simulink library "DQN_Lib"  (R2023b)
settings: Solver=VariableStepAuto  StartTime=0.0  StopTime=10.0  RelTol=1e-3
undefined symbols (not defined in the file): ACDC3, HRM, La, N, R, Ra, sps_AC, SYS, Ts, Ts_dqn, Ts_Power, w, Ws
libraries: DQN_Lib_bak x7
(part 1 of 3)
settings Model: Creator=Robert  LastModifiedBy=rober
settings DebuggingCC: UnconnectedInputMsg=warning  UnconnectedOutputMsg=warning  UnconnectedLineMsg=warning
settings ModelReferenceCC: EnableRefExpFcnMdlSchedulingChecks=on
settings RTWCC: DLArmComputeVersion=19.05

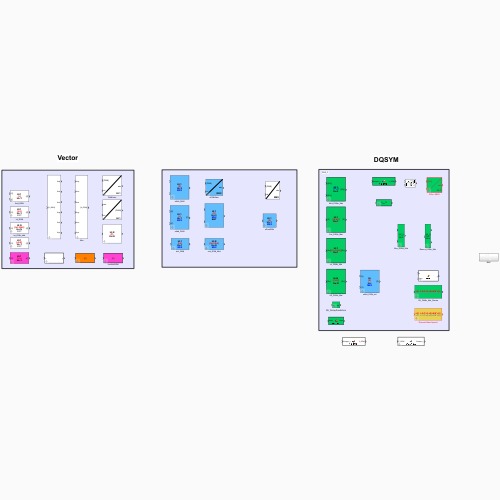
[thumbnail: Simulink's stored preview of the top-level diagram]
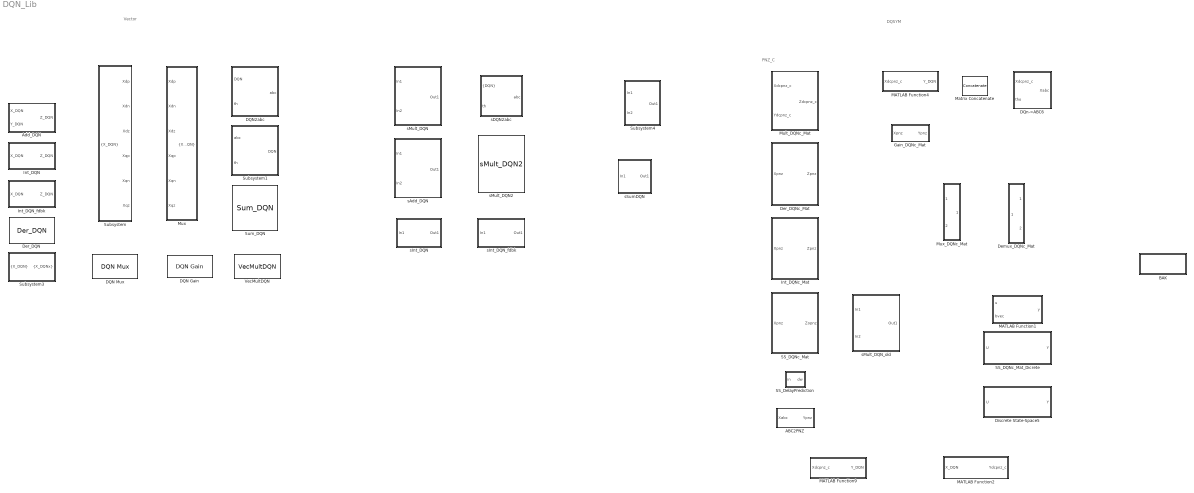
== system DQN_Lib ==
  note: PNZ_C
  note: DQSYM
  note: Vector
  ABC2PNZ : MATLAB Function  TreatAsAtomicUnit=on  SystemSampleTime=Ts
  Add_DQN : Subsystem  mask{HrmOrd=1, chkHrmLst=off, HrmLst=[1]}
      mask prompts: HrmOrd "Harmonic order:"; chkHrmLst "Only specific harmonics"; HrmLst "Harmonic list:"
      mask Callback chkHrmLst:
      | EMT = get_param(gcb,'chkHrmLst');
      | 
      | if(strcmp(EMT,'on'))
      |    set_param(gcb,'MaskVisibilities',{'on','on','on'});
      | else
      |    set_param(gcb,'MaskVisibilities',{'on','on','off'});
      | end
      mask Display:
      | %plot([0 1])
      | port_label('input',1,'{X}');
      | port_label('input',2,'{Y}');
      | port_label('output',1,'{Z}');
      | 
      | 
      | 
      | harm = get_param(gcb, 'HrmOrd');
      | disp(['{\color{black}\bf\fontsize{12}Hi:',(harm),'}',newline,'{\color{red}\bf\fontsize{12}\{+\}}',newline,'{\color{black}\bf\fontsize{12}Ho:',(harm),'}'], 'texmode','on');
  BAK : Subsystem
  DQN Gain : DQN_Lib_bak/DQN Gain  H=1  Rvec=[]
  DQN Mux : DQN_Lib_bak/DQN Mux  N=1
  DQN2abc : Subsystem  mask{HrmOrd=1}
      mask prompts: HrmOrd "Harmonic order:"
      mask Display:
      | plot([0 1], [0,1])
      | port_label('input',1,'{DQN}');
      | port_label('input',2,'wt');
      | port_label('output',1,'abc');
      | 
      | 
      | 
      | harm = get_param(gcb, 'HrmOrd');
      | %disp([newline,'{\bf\fontsize{12}H=',harm,'}'], 'texmode','on');
      | text(.95,.05,[newline,'{\bf\fontsize{12}H=',harm,'}'], 'horizontalAlignment', 'right', 'verticalAlignment','bottom','texmode','on')
  DQn->ABC6 : MATLAB Function  TreatAsAtomicUnit=on  mask{N=1}
      mask prompts: N "Harmonic order:"
  Demux_DQNc_Mat : Subsystem  mask{nrOut=2}
      mask prompts: nrOut "Number of outputs [{C}]"
      mask init:
      | if(isempty(nrOut))
      |     Simulink.SubSystem.deleteContents(gcb);
      | else
      | 
      |     IndexOptionArray = cell(2,1);
      |     IndexOptionArray(1) = {'Select all'           };
      |     IndexOptionArray(2) = {'Index vector (dialog)'};
      | 
      |     PortHandles = get_param(gcb,'PortHandles');
      | 
      |     lenOut = length(PortHandles.Outport);
      | 
      |     if(nrOut ~= lenOut) % Important to avoid reinitialization of the block!
      | 
      |         Simulink.SubSystem.deleteContents(gcb);
      | 
      |         add_block('built-in/Inport',[gcb,strcat('/In',num2str(1))]);
      |         set_param([gcb,strcat('/In',num2str(1))],'position' , [50,65+1*50,90,85+1*50]);
      | 
      |         for i = 1 : nrOut
      |             add_block('simulink/Signal Routing/Selector',[gcb,strcat('/Sel',num2str(i))],...
      |                 'IndexOptionArray',IndexOptionArray,...
      |                 'NumberOfDimensions','2',...
      |                 'IndexOptions','Index vector (dialog),Select all',...
      |                 'Indices',strcat(num2str((i-1)*3+1),':',num2str((i-1)*3+3),', 1') ...
      |                 );
      |             set_param([gcb,strcat('/Sel',num2str(i))],'position' , [450,65+i*50,490,85+i*50])
      | 
      | 
      |             add_block('built-in/Outport',[gcb,strcat('/Out',num2str(i))]);
      |             set_param([gcb,strcat('/Out',num2str(i))],'position' , [750,65+i*50,790,85+i*50]);
      | 
      |             add_line(gcb,strcat('In',num2str(1),'/1'),  strcat('Sel',num2str(i),'/1'),'autorouting','on');
      |             add_line(gcb,strcat('Sel',num2str(i),'/1'), strcat('Out',num2str(i),'/1'),'autorouting','on');
      |         end
      | 
      |     end
      | 
      | end
      mask Display: disp(['{\color{red}\bf\fontsize{12}} [\{X_C\}]',newline,' DE-',newline,' MUX'], 'texmode','on');
  Der_DQN : DQN_Lib_bak/Der_DQN  HrmOrd=1  FreqRad=2*pi*50  Ts=0  EMT=on  sw_soft=on  chkHrmLst=off  HrmLst=[1]
  Der_DQNc_Mat : MATLAB Function  TreatAsAtomicUnit=on  mask{Ts=50e-6, N=1, w=2*pi*50, EMT=on, sw_soft=on}
      mask prompts: Ts "Time step (s):"; N "Harmonic order:"; w "Angular frequency [1/rad]:"; sw_soft "Soft start"
  Discrete State-Space5 : Subsystem  mask{A=sps_AC.A, B=sps_AC.B, C=sps_AC.C, D=sps_AC.D, InitVec=sps_AC.x0, dt=Ts_Power, DQSYM=on, N=HRM, Ws=w}
      mask prompts: InitVec "Initial condition:"; dt "Time step (s):"; N "Harmonic number:"; Ws "Angular frequency (1/rad):"
      mask init:
      | % I = eye(size(A,1));
      | % INVR = I/(I-A*dt/2);
      | % Ad1 = INVR*(I+A*dt/2);
      | % Bd1 = INVR*B*dt/2;
      | % Cd1 = C*Ad1;
      | % Dd11 = C*INVR*B*dt/2+D;
      | % Dd12 = C*INVR*B*dt/2;
      | 
      |     I = eye(size(A,1));
      |     INVR = I/(I-A*dt/2);
      |     Ad1 = INVR*(I+A*dt/2);
      |     Bd1 = INVR*B;
      |     Cd1 = C*INVR*dt;
      |     Dd1 = Cd1*B/2 + D;
      | 
      | DQSYM = get_param(gcb,'DQSYM');
      | 
      | comp = 0;
      | 
      | if(strcmp(DQSYM,'on'))
      | 
      | %Calculating the PNZ matrices
      | 
      |     a = -0.5+0.866i;
      |     a2 = -0.5-0.866i;
      |     Sas = [1,a,a2;1,a2,a;1,1,1]/3;
      | 
      |     arows = size(Ad1,1)/3; %signal size
      |     acols = size(Ad1,2)/3; %signal size
      | 
      |     brows = size(Bd1,1)/3; %signal size
      |     bcols = size(Bd1,2)/3; %signal size
      | 
      |     crows = size(Cd1,1)/3; %signal size
      |     ccols = size(Cd1,2)/3; %signal size
      | 
      |     d1rows = size(Dd1,1)/3; %signal size
      |     d1cols = size(Dd1,2)/3; %signal size
      | 
      |     %%%%%%%%%%%%%%%%%%%%%%% Check for inconsistencies  %%%%%%%%%%%%%%%%%%%%%%%
      | 
      |     szMatA = size(A,1);
      |     iL = eye(szMatA);
      |     szMatiL = size(iL,1);
      | 
      |     if(szMatiL ~= szMatA || size(A,1) ~= size(A,2) || size(iL,1) ~= size(iL,2))
      |         error('[Int_DQN_Mat/swFeedback] check matrix A size!');
      |     end
      | 
      |     if(arows ~= brows || acols ~= ccols || crows ~= d1rows || bcols ~= d1cols)
      |         error('[Int_DQN_Mat/Initialize] the sizes of the state-space matrices!');
      |     end
      | 
      |     %%%%%%%%%%%%%%%%%%%%%%%%%%%%%%%%%%%%%%%%%%%%%%%%%%%%%%%%%%%%%%%
      | 
      | 
      |     %%%%%%%%%%%%%%%%%%%%%%% A --> Bpnz %%%%%%%%%%%%%%%%%%%%%%%
      |     Adc = complex(zeros(3*arows,3*acols));
      | 
      |     for i = 1 : arows
      |         for j = 1 : acols
      |             Adc((1:3) + (i-1)*3,(1:3) + (j-1)*3) = Sas*Ad1((1:3) + (i-1)*3,(1:3) + (j-1)*3)/Sas;
      |             %Adc((1:3) + (i-1)*3,(1:3) + (j-1)*3) = diag(diag(real(Adc((1:3) + (i-1)*3,(1:3) + (j-1)*3))));
      |             %Adc((1:3) + (i-1)*3,(1:3) + (j-1)*3) = diag(diag((Adc((1:3) + (i-1)*3,(1:3) + (j-1)*3))));
      | 
      |         end
      |     end
      |     %%%%%%%%%%%%%%%%%%%%%%%%%%%%%%%%%%%%%%%%%%%%%%%%%%%%%%%%%%%%%%%
      | 
      |     %%%%%%%%%%%%%%%%%%%%%%% B --> Bpnz %%%%%%%%%%%%%%%%%%%%%%%
      | 
      |     Bdc = complex(zeros(3*brows,3*bcols));
      | 
      |     for i = 1 : brows
      |         for j = 1 : bcols
      |             Bdc((1:3) + (i-1)*3,(1:3) + (j-1)*3) = Sas*Bd1((1:3) + (i-1)*3,(1:3) + (j-1)*3)/Sas;
      |             %Bdc((1:3) + (i-1)*3,(1:3) + (j-1)*3) = diag(diag(real(Bdc((1:3) + (i-1)*3,(1:3) + (j-1)*3))));
      |             %Bdc((1:3) + (i-1)*3,(1:3) + (j-1)*3) = diag(diag((Bdc((1:3) + (i-1)*3,(1:3) + (j-1)*3))));
      | 
      |         end
      |     end
      |     %%%%%%%%%%%%%%%%%%%%%%%%%%%%%%%%%%%%%%%%%%%%%%%%%%%%%%%%%%%%%%%
      | 
      |     %%%%%%%%%%%%%%%%%%%%%%% C --> Cpnz %%%%%%%%%%%%%%%%%%%%%%%
      | 
      |     Cdc = complex(zeros(3*crows,3*ccols));
      | 
      |     for i = 1 : crows
      |         for j = 1 : ccols
      |             Cdc((1:3) + (i-1)*3,(1:3) + (j-1)*3) = Sas*Cd1((1:3) + (i-1)*3,(1:3) + (j-1)*3)/Sas;
      |             %Cdc((1:3) + (i-1)*3,(1:3) + (j-1)*3) = diag(diag(real(Cdc((1:3) + (i-1)*3,(1:3) + (j-1)*3))));
      |             %Cdc((1:3) + (i-1)*3,(1:3) + (j-1)*3) = diag(diag((Cdc((1:3) + (i-1)*3,(1:3) + (j-1)*3))));
      |         end
      |     end
      |     %%%%%%%%%%%%%%%%%%%%%%%%%%%%%%%%%%%%%%%%%%%%%%%%%%%%%%%%%%%%%%%
      | 
      |     
      |     %%%%%%%%%%%%%%%%%%%%%%% D1 --> Cpnz %%%%%%%%%%%%%%%%%%%%%%%
      | 
      |     Ddc = complex(zeros(3*d1rows,3*d1cols));
      | 
      |     for i = 1 : d1rows
      |         for j = 1 : d1cols
      |             Ddc((1:3) + (i-1)*3,(1:3) + (j-1)*3) = Sas*Dd1((1:3) + (i-1)*3,(1:3) + (j-1)*3)/Sas;
      |             %Ddc1((1:3) + (i-1)*3,(1:3) + (j-1)*3) = diag(diag(real(Ddc1((1:3) + (i-1)*3,(1:3) + (j-1)*3))));
      |             %Ddc((1:3) + (i-1)*3,(1:3) + (j-1)*3) = diag(diag((Ddc((1:3) + (i-1)*3,(1:3) + (j-1)*3))));
      |         end
      |     end
      |     %%%%%%%%%%%%%%%%%%%%%%%%%%%%%%%%%%%%%%%%%%%%%%%%%%%%%%%%%%%%%%%
      | 
      |     Adc(abs(Adc)<2*eps) = 0;
      |     Bdc(abs(Bdc)<2*eps) = 0;
      |     Cdc(abs(Cdc)<2*eps) = 0;
      |     Ddc(abs(Ddc)<2*eps) = 0;
      | 
      |     InitVec_c = complex(zeros(brows*3,N+1));
      | 
      | 
      |     if(~isempty(InitVec))
      |         if(mod(numel(InitVec),3)~=0) 
      |             warning('[SS_DQNc_Mat] InitVec with wrong size --> needs to be a multiple of 3!'); 
      | 
      |         else
      |             for k = 1 : numel(InitVec)/3
      |                 InitVec_c((k-1)*3+1:(k-1)*3+3,1) = Sas*InitVec((k-1)*3+1:(k-1)*3+3)*exp(+1i*Ws*dt);
      |             end
      |         end
      |     end
      | 
      |     InitVec = InitVec_c;
      | 
      | 
      |     Ad1 = Adc;
      |     Bd1 = Bdc;
      |     Cd1 = Cdc;
      |     Dd1 = Ddc;
      | 
      |     comp = -1i*Ws*dt;
      | 
      | end
      settings: LibrarySourceBlock=|
      | spsSynchronousMachineModel/Discrete robust/State Space Model/Discretize
      | BE or Tustin
      mask Callback DQSYM:
      | EMT = get_param(gcb,'DQSYM');
      | 
      | if(strcmp(EMT,'on'))
      |    set_param(gcb,'MaskVisibilities',{'on','on','on','on','on','on','on','on','on'});
      | else
      |    set_param(gcb,'MaskVisibilities',{'on','on','on','on','on','on','on','off','off'});
      | end
      mask Display: disp(['{\color{red}\bf\fontsize{12}x(t) = Ad*x(t-dt)+Bd*u(t)}',newline,'{\color{gray}\bf\fontsize{12}y(t) = Cd*x(t-dt)+Dd*u(t)}'], 'texmode','on');
  Gain_DQNc_Mat : MATLAB Function  TreatAsAtomicUnit=on  mask{Rabc=[R zeros(3,3); zeros(3,3) R], HRM=N, chkInv=off}
      mask prompts: Rabc "Line matrix [3x3]:"; HRM "Harmonic order:"; chkInv "Invert"
  Int_DQN : Subsystem  mask{HrmOrd=1, FreqRad=2*pi*50, TimeStep=50e-6, Init=zeros(1,6), EMT=on, chkHrmLst=off, HrmLst=[1]}
      mask prompts: HrmOrd "Harmonic order:"; FreqRad "Angular frequency (rad/s);"; TimeStep "Time step (s):"; Init "DC init [1x6]:"; EMT "Enable EMT"; chkHrmLst "Only specific harmonics"; HrmLst "Harmonic list:"
      mask Callback chkHrmLst:
      | EMT = get_param(gcb,'chkHrmLst');
      | 
      | if(strcmp(EMT,'on'))
      |    set_param(gcb,'MaskVisibilities',{'on','on','on','on','on','on','on'});
      | else
      |    set_param(gcb,'MaskVisibilities',{'on','on','on','on','on','on','off'});
      | end
      mask Display:
      | %plot([0 1])
      | port_label('input',1,'{X}');
      | port_label('output',1,'{Z}');
      | 
      | harm = get_param(gcb, 'HrmOrd');
      | 
      | if(numel(get_param(gcb, 'EMT'))==2)
      |     disp(['{\color{black}\bf\fontsize{12}Hi:',(harm),'}',newline,'{\color{red}\bf\fontsize{12}\{Int\}}',newline,'{\color{black}\bf\fontsize{12}Ho:',(harm),'}',newline,'{\color{gray}\bf\fontsize{12}EMT}'], 'texmode','on');
      | else
      |     disp(['{\color{black}\bf\fontsize{12}Hi:',(harm),'}',newline,'{\color{red}\bf\fontsize{12}\{Int\}}',newline,'{\color{black}\bf\fontsize{12}Ho:',(harm),'}'], 'texmode','on');
      | end
  Int_DQN_fdbk : Subsystem  mask{HrmOrd=N, FreqRad=Ws, TimeStep=Ts_dqn, swFeed=on, R=Ra, iL=1/La}
      mask prompts: HrmOrd "Harmonic order:"; FreqRad "Angular frequency (rad/s);"; TimeStep "Time step (s):"; swFeed "Enable feedback"; R "Feedback parameter (Kr):"; iL "Integrator parameter (Kl):"
      mask Callback swFeed:
      | EMT = get_param(gcb,'swFeed');
      | 
      | if(strcmp(EMT,'on'))
      |    set_param(gcb,'MaskVisibilities',{'on','on','on','on','on','on'});
      | else
      |    set_param(gcb,'MaskVisibilities',{'on','on','on','on','off','off'});
      | end
      mask Display:
      | %plot([0 1])
      | port_label('input',1,'{X}');
      | port_label('output',1,'{Z}');
      | 
      | harm = get_param(gcb, 'HrmOrd');
      | disp(['{\color{black}\bf\fontsize{12}Hi:',(harm),'}',newline,'{\color{red}\bf\fontsize{12}\{Int-fdbk\}}',newline,'{\color{black}\bf\fontsize{12}Ho:',(harm),'}',newline,'{\color{gray}\bf\fontsize{12}EMT}'], 'texmode','on');
  Int_DQNc_Mat : MATLAB Function  TreatAsAtomicUnit=on  mask{N=1, dt=50e-6, w=2*pi*50, InitInt=zeros(3,1), swFeed=on, R=eye(3), iL=eye(3)}
      mask prompts: N "Order number:"; dt "Time step (s):"; w "Angular frequency (1/rad):"; InitInt "Initial conditions DC [3x1]:"; swFeed "Enable feedback"; R "Feedback parameter (Kr {abc}):"; iL "Feedback parameter (Ki {abc}):"
  MATLAB Function1 : MATLAB Function  TreatAsAtomicUnit=on  mask{Ad=ACDC3.Adiscrete, Bd=ACDC3.Bdiscrete, Cd=ACDC3.Cdiscrete, Dd=ACDC3.Ddiscrete, InitVec=ACDC3.x0, dt=Ts_Power, nsw=6}
      mask prompts: Ad "A"; Bd "B"; Cd "C"; Dd "D"; InitVec "Initial values:"; dt "Time step (s):"; nsw "Number of switches:"
  MATLAB Function2 : MATLAB Function  TreatAsAtomicUnit=on  mask{N=HRM}
      mask prompts: N "Harmonic order:"
  MATLAB Function4 : MATLAB Function  TreatAsAtomicUnit=on
  MATLAB Function9 : MATLAB Function  TreatAsAtomicUnit=on
  Matrix Concatenate : Concatenate  Mode=Multidimensional array  ConcatenateDimension=2
  Mult_DQNc_Mat : MATLAB Function  TreatAsAtomicUnit=on  mask{N=1, HrmDbl=on}
      mask prompts: N "Harmonic order:"; HrmDbl "Double Harmonic"
  Mux : Subsystem  mask{N=1}
      mask prompts: N "Harmonic order:"
  Mux_DQNc_Mat : Subsystem  mask{nrInp=2}
      mask prompts: nrInp "Number of inputs [{C}]"
      mask init:
      | %blocks = find_system(gcb,'LookUnderMasks','on','FollowLinks','on')
      | %set_param(gcb, 'MaskSelfModifiable', 'on');
      | 
      | % if(SSM == [])
      | %     Simulink.SubSystem.deleteContents(gcb);
      | % else
      | 
      | if(isempty(nrInp))
      |     Simulink.SubSystem.deleteContents(gcb);
      | else
      | 
      |     nrOut = 1;
      | 
      | 
      | PortHandles = get_param(gcb,'PortHandles');
      | lenInp = length(PortHandles.Inport);
      | lenOut = length(PortHandles.Inport);
      | 
      | if(nrInp ~= lenInp)
      |     %disp('ENTERED')
      |     Simulink.SubSystem.deleteContents(gcb);
      | %     add_block('simulink/Continuous/State-Space', [gcb,'/ss_block'], 'A','SS.A', 'B','SS.B', 'C','SS.C', 'D','SS.D', 'X0','X0')
      | %     set_param([gcb,'/ss_block'],'position' , [350,100,450,150])
      | 
      | 
      | 
      |         add_block('simulink/Math Operations/Matrix Concatenate',[gcb,'/Mux'], 'NumInputs',num2str(nrInp), 'ConcatenateDimension',num2str(1));
      |         set_param([gcb,'/Mux'],'position' , [200,100,250,100+nrInp*50])
      |         
      | %         add_block('built-in/Demux',[gcb,'/Demux'], 'Outputs',num2str(nrOut));
      | %         set_param([gcb,'/Demux'],'position' , [500,100,550,100+nrOut*50])
      | 
      | 
      |         for i = 1 : nrInp
      |             add_block('built-in/Inport',[gcb,strcat('/In',num2str(i))]);
      |             set_param([gcb,strcat('/In',num2str(i))],'position' , [50,65+i*50,90,85+i*50]);
      |             add_line(gcb,strcat('In',num2str(i),'/1'),strcat('Mux/',num2str(i)),'autorouting','on');
      |         end
      | 
      |         for i = 1 : nrOut
      |             add_block('built-in/Outport',[gcb,strcat('/Out',num2str(i))]);
      |             set_param([gcb,strcat('/Out',num2str(i))],'position' , [750,65+i*50,790,85+i*50]);
      |             add_line(gcb,strcat('Mux/',num2str(i)), strcat('Out',num2str(i),'/1'),'autorouting','on');
      |         end
      | 
      | 
      | %     add_line(gcb, 'Mux/1', 'ss_block/1')
      | %     add_line(gcb, 'ss_block/1', 'Demux/1')
      | 
      | end
      | 
      | end
      mask Display: disp(['{\color{red}\bf\fontsize{12}} [\{X_C\}]',newline,' MUX'], 'texmode','on');
  SS_DQNc_Mat : MATLAB Function  TreatAsAtomicUnit=on  mask{N=N, A=[], B=[], C=[], D=[], dt=50e-6, w=2*pi*50, x0=[], stNames=[]}
      mask prompts: N "Order number:"; dt "Time step (s):"; w "Angular frequency (1/rad):"; x0 "Initial conditions:"; stNames "State names:"
      mask init:
      | szA = size(A,1);
      | 
      | [~, I] = sort(stNames(1:szA));
      | 
      | 
      | A = A(I,I);
      | B = B(I,:);
      | C = -C(:,I);
      | D = D;
      | 
      | x0 = x0(I,:);
  SS_DQNc_Mat_Dicrete : Subsystem  mask{A=SYS.A, B=SYS.B, C=SYS.C, D=SYS.D, InitVec=SYS.x0, dt=Ts, N=N, Ws=2*pi*50}
      mask prompts: InitVec "Initial condition:"; dt "Time step (s):"; N "Harmonic order:"; Ws "Angular frequency (rad/s):"
      mask init:
      | I = eye(size(A,1));
      |     
      |     INVR = I/(I-A*dt/2);
      |     
      |     Ad = INVR*(I+A*dt/2);
      |     
      |     Bd = INVR*B;
      |     
      |     Cd = C*INVR*dt;
      |     
      |     Dd = Cd*B/2;
      | 
      |     dt2 = dt/2;
      | 
      |     a = -0.5+0.866i;
      |     a2 = -0.5-0.866i;
      |     Sas = [1,a,a2;1,a2,a;1,1,1]/3;
      | 
      |     arows = size(Ad,1)/3; %signal size
      |     acols = size(Ad,2)/3; %signal size
      | 
      |     brows = size(Bd,1)/3; %signal size
      |     bcols = size(Bd,2)/3; %signal size
      | 
      |     crows = size(Cd,1)/3; %signal size
      |     ccols = size(Cd,2)/3; %signal size
      | 
      |     drows = size(Dd,1)/3; %signal size
      |     dcols = size(Dd,2)/3; %signal size
      | 
      |     %%%%%%%%%%%%%%%%%%%%%%% Check for inconsistencies  %%%%%%%%%%%%%%%%%%%%%%%
      | 
      |     szMatA = size(A,1);
      |     iL = eye(szMatA);
      |     szMatiL = size(iL,1);
      | 
      |     if(szMatiL ~= szMatA || size(A,1) ~= size(A,2) || size(iL,1) ~= size(iL,2))
      |         error('[Int_DQN_Mat/swFeedback] check matrix A size!');
      |     end
      | 
      |     if(arows ~= brows || acols ~= ccols || crows ~= drows || bcols ~= dcols)
      |         error('[Int_DQN_Mat/Initialize] the sizes of the state-space matrices!');
      |     end
      | 
      |     %%%%%%%%%%%%%%%%%%%%%%%%%%%%%%%%%%%%%%%%%%%%%%%%%%%%%%%%%%%%%%%
      | 
      |     %%%%%%%%%%%%%%%%%%%%%%% A --> Bpnz %%%%%%%%%%%%%%%%%%%%%%%
      |     Adc = complex(zeros(3*arows,3*acols));
      | 
      |     for i = 1 : arows
      |         for j = 1 : acols
      |             Adc((1:3) + (i-1)*3,(1:3) + (j-1)*3) = Sas*Ad((1:3) + (i-1)*3,(1:3) + (j-1)*3)/Sas;
      |             %Adc((1:3) + (i-1)*3,(1:3) + (j-1)*3) = diag(diag(real(Adc((1:3) + (i-1)*3,(1:3) + (j-1)*3))));
      |         end
      |     end
      |     %%%%%%%%%%%%%%%%%%%%%%%%%%%%%%%%%%%%%%%%%%%%%%%%%%%%%%%%%%%%%%%
      | 
      |     %%%%%%%%%%%%%%%%%%%%%%% B --> Bpnz %%%%%%%%%%%%%%%%%%%%%%%
      | 
      |     Bdc = complex(zeros(3*brows,3*bcols));
      | 
      |     for i = 1 : brows
      |         for j = 1 : bcols
      |             Bdc((1:3) + (i-1)*3,(1:3) + (j-1)*3) = Sas*Bd((1:3) + (i-1)*3,(1:3) + (j-1)*3)/Sas;
      |             %Bdc((1:3) + (i-1)*3,(1:3) + (j-1)*3) = diag(diag(real(Bdc((1:3) + (i-1)*3,(1:3) + (j-1)*3))));
      |         end
      |     end
      |     %%%%%%%%%%%%%%%%%%%%%%%%%%%%%%%%%%%%%%%%%%%%%%%%%%%%%%%%%%%%%%%
      | 
      |     %%%%%%%%%%%%%%%%%%%%%%% C --> Cpnz %%%%%%%%%%%%%%%%%%%%%%%
      | 
      |     Cdc = complex(zeros(3*crows,3*ccols));
      | 
      |     for i = 1 : crows
      |         for j = 1 : ccols
      |             Cdc((1:3) + (i-1)*3,(1:3) + (j-1)*3) = Sas*Cd((1:3) + (i-1)*3,(1:3) + (j-1)*3)/Sas;
      |             %Cdc((1:3) + (i-1)*3,(1:3) + (j-1)*3) = diag(diag(real(Cdc((1:3) + (i-1)*3,(1:3) + (j-1)*3))));
      |         end
      |     end
      |     %%%%%%%%%%%%%%%%%%%%%%%%%%%%%%%%%%%%%%%%%%%%%%%%%%%%%%%%%%%%%%%
      | 
      |     %%%%%%%%%%%%%%%%%%%%%%% C --> Cpnz %%%%%%%%%%%%%%%%%%%%%%%
      | 
      |     Ddc = complex(zeros(3*drows,3*dcols));
      | 
      |     for i = 1 : drows
      |         for j = 1 : dcols
      |             Ddc((1:3) + (i-1)*3,(1:3) + (j-1)*3) = Sas*Dd((1:3) + (i-1)*3,(1:3) + (j-1)*3)/Sas;
      |             %Ddc((1:3) + (i-1)*3,(1:3) + (j-1)*3) = diag(diag(real(Ddc((1:3) + (i-1)*3,(1:3) + (j-1)*3))));
      |         end
      |     end
      |     %%%%%%%%%%%%%%%%%%%%%%%%%%%%%%%%%%%%%%%%%%%%%%%%%%%%%%%%%%%%%%%
      | 
      | 
      | 
      |     Adc(abs(Adc)<2*eps) = 0;
      |     Bdc(abs(Bdc)<2*eps) = 0;
      |     Cdc(abs(Cdc)<2*eps) = 0;
      |     Ddc(abs(Ddc)<2*eps) = 0;
      | 
      |     % Adc = real(Adc);
      |     % Bdc = real(Bdc);
      |     % Cdc = real(Cdc);
      |     % Ddc = real(Ddc);
      | 
      | 
      |     InitVec_c = complex(zeros(brows*3,N+1));
      | 
      | 
      |     if(~isempty(InitVec))
      |         if(mod(numel(InitVec),3)~=0) error('[SS_DQNc_Mat] InitVec with wrong size --> needs to be a multiple of 3!'); end
      | 
      |         for k = 1 : numel(InitVec)/3
      |             InitVec_c((k-1)*3+1:(k-1)*3+3,1) = Sas*InitVec((k-1)*3+1:(k-1)*3+3);
      |         end
      |     end
      settings: LibrarySourceBlock=|
      | spsSynchronousMachineModel/Discrete robust/State Space Model/Discretize
      | BE or Tustin
      mask Display: disp(['{\color{red}\bf\fontsize{12}x(t) = Ad*x(t-dt)+Bd*u(t)}',newline,'{\color{gray}\bf\fontsize{12}y(t) = Cd*x(t-dt)+Dd*u(t)}'], 'texmode','on');
  SS_DelayPrediction : Subsystem  mask{N=1, Ts=50e-6, x0=zeros(3,1)}
      mask prompts: N "Order number:"; Ts "Time step (s):"; x0 "Initial conditions (x0):"
      mask init:
      | a = -0.5+0.866i;
      | a2 = -0.5-0.866i;
      | Sas = [1,a,a2;1,a2,a;1,1,1]/3;
      | 
      | Zpnz_old = complex(zeros(size(x0,1),N+1));
      | 
      | if(~isempty(x0))
      | 
      |     if(mod(numel(x0),3)~=0) error('[Delay predictor] x0 vector with wrong size --> needs to be a multiple of 3!'); end
      | 
      |     for k = 1 : numel(x0)/3
      |         Zpnz_old((k-1)*3+1:(k-1)*3+3,1) = Sas*x0((k-1)*3+1:(k-1)*3+3);
      |     end
      | end
  Subsystem : Subsystem  mask{N=1}
      mask prompts: N "Harmonic order:"
  Subsystem1 : Subsystem  mask{HrmOrd=1, Freq=0, Ts=50e-6}
      mask prompts: HrmOrd "Harmonic order:"; Freq "Frequency (Hz):"; Ts "Sample time (s):"
      mask Display:
      | plot([0 1], [0,1])
      | port_label('input',1,'abc');
      | port_label('input',2,'wt');
      | port_label('output',1,'{DQN}');
      | 
      | 
      | 
      | harm = get_param(gcb, 'HrmOrd');
      | %disp([newline,'{\bf\fontsize{12}H=',harm,'}'], 'texmode','on');
      | text(.95,.05,[newline,'{\bf\fontsize{12}H=',harm,'}'], 'horizontalAlignment', 'right', 'verticalAlignment','bottom','texmode','on')
  Subsystem3 : Subsystem  mask{HOI=1, HOO=1}
      mask prompts: HOI "Input harmonic order:"; HOO "Output harmonic order:"
      mask Display:
      | %plot([0 1])
      | port_label('input',1,'{X}');
      | port_label('output',1,'{Y}');
      | 
      | 
      | 
      | HOI = get_param(gcb, 'HOI');
      | HOO = get_param(gcb, 'HOO');
      | disp(['{\color{black}\bf\fontsize{12}Hi:',(HOI),'}',newline,'{\color{red}\bf\fontsize{12}Trim}',newline,'{\color{black}\bf\fontsize{12}Ho:',(HOO),'}'], 'texmode','on');
  Subsystem4 : Subsystem
      mask Display:
      | plot([0 1], [0,1])
      | port_label('input',1,'{DQN}');
      | port_label('input',2,'wt');
      | port_label('output',1,'abc');
      | 
      | text(.95,.05,[newline,'{\bf\fontsize{12}MEX}'], 'horizontalAlignment', 'right', 'verticalAlignment','bottom','texmode','on')
  Sum_DQN : DQN_Lib_bak/Sum_DQN  HrmOrd=N
  VecMultDQN : DQN_Lib_bak/VecMultDQN  H=1  R=[]  chkInv=off
  sAdd_DQN : Subsystem  mask{HRM=1}
      mask prompts: HRM "Harmonic order:"
      mask Display:
      | %plot([0 1])
      | port_label('input',1,'{X}');
      | port_label('input',2,'{Y}');
      | port_label('output',1,'{Z}');
      | 
      | 
      | 
      | %harm = (get_param(gcb, 'HRM'));
      | %disp(['{\color{black}\bf\fontsize{12}Hi:',num2str(harm),'}',newline,'{\color{red}\bf\fontsize{12}\{+\}}',newline,'{\color{black}\bf\fontsize{12}Ho:',num2str(harm),newline,'{\color{blue}\bf\fontsize{12}MEX}','}'], 'texmode','on');
      | harm = get_param(gcb, 'HRM');
      | disp(['{\color{black}\bf\fontsize{12}Hi:',(harm),'}',newline,'{\color{red}\bf\fontsize{12}\{+\}}',newline,'{\color{black}\bf\fontsize{12}Ho:',(harm),newline,'{\color{blue}\bf\fontsize{12}MEX}','}'], 'texmode','on');
  sDQN2abc : Subsystem  mask{HRM=1}
      mask prompts: HRM "Harmonic order:"
      mask Display:
      | plot([0 1], [0,1])
      | port_label('input',1,'{DQN}');
      | port_label('input',2,'wt');
      | port_label('output',1,'abc');
      | 
      | text(.95,.05,[newline,'{\bf\fontsize{12}MEX}'], 'horizontalAlignment', 'right', 'verticalAlignment','bottom','texmode','on')
  sInt_DQN : Subsystem  mask{HRM=1, Ws=2*pi*50, Ts=50e-6, HrmSeq=off}
      mask prompts: HRM "Harmonic order:"; Ws "Angular frequency (1/rad):"; Ts "Time step (s):"; HrmSeq "Pos. odd / neg. even harmonics (1p, 2n, 3p...)"
      mask Display:
      | %plot([0 1])
      | %port_label('input',1,'{X}');
      | %port_label('output',1,'{Z}');
      | 
      | port_label('input',1,'');
      | port_label('output',1,'');
      | 
      | harm = get_param(gcb, 'HRM');
      | 
      | disp(['{\color{black}\bf\fontsize{12}Hi:',(harm),'}',newline,'{\color{red}\bf\fontsize{12}\{Int\}}',newline,'{\color{black}\bf\fontsize{12}Ho:',(harm),'}',newline,'{\color{blue}\bf\fontsize{12}MEX}'], 'texmode','on');
  sInt_DQN_fdbk : Subsystem  mask{HRM=N, Ws=Ws, Ts=Ts, HrmSeq=off, swFeed=off, R=1, iL=1}
      mask prompts: HRM "Harmonic order:"; Ws "Angular frequency (1/rad):"; Ts "Time step (s):"; HrmSeq "Pos. odd / neg. even harmonics (1p, 2n, 3p...)"; swFeed "Enable feedback"; R "Feedback parameter (Kr):"; iL "Integrator parameter (Ki):"
      mask Callback swFeed:
      | EMT = get_param(gcb,'swFeed');
      | 
      | if(strcmp(EMT,'on'))
      |    set_param(gcb,'MaskVisibilities',{'on','on','on','on','on','on','on'});
      | else
      |    set_param(gcb,'MaskVisibilities',{'on','on','on','on','on','off','off'});
      | end
      mask Display:
      | %plot([0 1])
      | %port_label('input',1,'{X}');
      | %port_label('output',1,'{Z}');
      | 
      | port_label('input',1,'');
      | port_label('output',1,'');
      | 
      | harm = get_param(gcb, 'HRM');
      | 
      | disp(['{\color{black}\bf\fontsize{12}Hi:',(harm),'}',newline,'{\color{red}\bf\fontsize{12}\{Int-fdbk\}}',newline,'{\color{black}\bf\fontsize{12}Ho:',(harm),'}',newline,'{\color{blue}\bf\fontsize{12}MEX}'], 'texmode','on');
  sMult_DQN : Subsystem  mask{HRM=1, HrmDbl=on, HrmSeq=off}
      mask prompts: HRM "Harmonic order:"; HrmDbl "Double harmonic"; HrmSeq "Pos. odd / neg. even harmonics (1p, 2n, 3p...)"
      mask init:
      | if(HrmDbl == 0 && HrmSeq == 0)
      |     HrmOpt = 0;
      | elseif(HrmDbl == 1 && HrmSeq == 0)
      |     HrmOpt = 1;
      | elseif(HrmDbl == 0 && HrmSeq == 1)
      |     HrmOpt = 2;
      | elseif(HrmDbl == 1 && HrmSeq == 1)
      |     HrmOpt = 3;
      | end
      mask Display:
      | %plot([0 1])
      | %port_label('input',1,'{X}');
      | %port_label('input',2,'{Y}');
      | %port_label('output',1,'{Z}');
      | 
      | port_label('input',1,'');
      | port_label('input',2,'');
      | port_label('output',1,'');
      | 
      | 
      | harm = str2num(get_param(gcb, 'HRM'));
      | HrmDbl = get_param(gcb, 'HrmDbl');
      | if(HrmDbl=="on")
      |     disp(['{\color{black}\bf\fontsize{12}Hi:',num2str(harm),'}',newline,'{\color{red}\bf\fontsize{12}\{X\}}',newline,'{\color{black}\bf\fontsize{12}Ho:',num2str(2*harm),newline,'{\color{blue}\bf\fontsize{12}MEX}','}'], 'texmode','on');
      | else
      |     disp(['{\color{black}\bf\fontsize{12}Hi:',num2str(harm),'}',newline,'{\color{red}\bf\fontsize{12}\{X\}}',newline,'{\color{black}\bf\fontsize{12}Ho:',num2str(harm),newline,'{\color{orange}\bf\fontsize{12}MEX}','}'], 'texmode','on');
      | end
      | 
      | %disp([newline,newline,newline,newline,newline,'{\color{black}\bf\fontsize{12}MEX}'],  'texmode','on');
      | 
      | 
      | 
      | %text(.95,.05,[newline,'{\bf\fontsize{12}H=',harm,'}'], 'horizontalAlignment', 'right', 'verticalAlignment','bottom','texmode','on')
  sMult_DQN2 : DQN_Lib_bak/sMult_DQN2  HRM=1  HrmDbl=on  selHrm=on  selMat=zeros(3,6)
  sMult_DQN_old : Subsystem  mask{HrmOrd=N, HrmDbl=on}
      mask prompts: HrmOrd "Harmonic order"; HrmDbl "Double harmonic?"
      mask Display:
      | %plot([0 1])
      | port_label('input',1,'{X}');
      | port_label('input',2,'{Y}');
      | port_label('output',1,'{Z}');
      | 
      | 
      | 
      | harm = str2num(get_param(gcb, 'HrmOrd'));
      | HrmDbl = get_param(gcb, 'HrmDbl');
      | if(HrmDbl=="on")
      |     disp(['{\color{black}\bf\fontsize{12}Hi:',num2str(harm),'}',newline,'{\color{red}\bf\fontsize{12}\{X\}}',newline,'{\color{black}\bf\fontsize{12}Ho:',num2str(2*harm),newline,'{\color{blue}\bf\fontsize{12}MEX}','}'], 'texmode','on');
      | else
      |     disp(['{\color{black}\bf\fontsize{12}Hi:',num2str(harm),'}',newline,'{\color{red}\bf\fontsize{12}\{X\}}',newline,'{\color{black}\bf\fontsize{12}Ho:',num2str(harm),newline,'{\color{orange}\bf\fontsize{12}MEX}','}'], 'texmode','on');
      | end
      | 
      | %disp([newline,newline,newline,newline,newline,'{\color{black}\bf\fontsize{12}MEX}'],  'texmode','on');
      | 
      | 
      | 
      | %text(.95,.05,[newline,'{\bf\fontsize{12}H=',harm,'}'], 'horizontalAlignment', 'right', 'verticalAlignment','bottom','texmode','on')
  sSumDQN : Subsystem  mask{HrmOrd=1}
      mask prompts: HrmOrd "Harmonic order:"
      mask Display:
      | %plot([0 1])
      | %port_label('input',1,'{X}');
      | %port_label('output',1,'{Z}');
      | 
      | port_label('input',1,'');
      | port_label('output',1,'');
      | 
      | harm = get_param(gcb, 'HrmOrd');
      | disp(['{\color{black}\bf\fontsize{12}Hi:',(harm),'}',newline,'{\color{red}\bf\fontsize{12}\{\Sigma\}}',newline,'{\color{black}\bf\fontsize{12}Ho:',(harm),'}',newline,'{\color{blue}\bf\fontsize{12}MEX}'], 'texmode','on');

== system DQN_Lib/Add_DQN ==
  X_DQN : Inport
  Y_DQN : Inport  Port=2
  Demux : Demux  Outputs=6
  Demux1 : Demux  Outputs=6
  MATLAB Function1 : MATLAB Function  TreatAsAtomicUnit=on  mask{N=HrmOrd, chkHrmLst=chkHrmLst, HrmLst=HrmLst}
      mask prompts: N "Harmonic order:"; chkHrmLst "Chosen harmonics"; HrmLst "Harmonic list:"
  Mux51 : Mux  Inputs=[(1)*HrmOrd+1,(1)*HrmOrd+1,(1)*HrmOrd+1,(1)*HrmOrd+1,(1)*HrmOrd+1,(1)*HrmOrd+1]
  Z_DQN : Outport
  wires:
  Demux1/6 -> MATLAB Function1/12(Yqz)
  Demux1/5 -> MATLAB Function1/11(Yqn)
  Demux1/4 -> MATLAB Function1/10(Yqp)
  Demux1/3 -> MATLAB Function1/9(Ydz)
  Demux1/2 -> MATLAB Function1/8(Ydn)
  Demux1/1 -> MATLAB Function1/7(Ydp)
  Demux/6 -> MATLAB Function1/6(Xqz)
  Demux/5 -> MATLAB Function1/5(Xqn)
  Demux/4 -> MATLAB Function1/4(Xqp)
  Demux/3 -> MATLAB Function1/3(Xdz)
  Demux/2 -> MATLAB Function1/2(Xdn)
  Demux/1 -> MATLAB Function1/1(Xdp)
  MATLAB Function1/6(Zqz) -> Mux51/6
  MATLAB Function1/5(Zqn) -> Mux51/5
  MATLAB Function1/1(Zdp) -> Mux51/1
  MATLAB Function1/4(Zqp) -> Mux51/4
  MATLAB Function1/2(Zdn) -> Mux51/2
  MATLAB Function1/3(Zdz) -> Mux51/3
  Mux51/1 -> Z_DQN/1
  Y_DQN/1 -> Demux1/1
  X_DQN/1 -> Demux/1

== system DQN_Lib/BAK ==
  Discrete State-Space : Subsystem  mask{A=1, B=1, C=1, D=1, InitVec=0, dt=50e-6}
      mask prompts: InitVec "Initial condition:"; dt "Time step (s):"
      mask init:
      | I = eye(size(A,1));
      | INVR = I/(I-A*dt/2);
      | Ad1 = INVR*(I+A*dt/2);
      | Bd1 = INVR*B*dt/2;
      | Cd1 = C*Ad1;
      | Dd11 = C*INVR*B*dt/2+D;
      | Dd12 = C*INVR*B*dt/2;
      settings: LibrarySourceBlock=|
      | spsSynchronousMachineModel/Discrete robust/State Space Model/Discretize
      | BE or Tustin
      mask Display: disp(['{\color{red}\bf\fontsize{12}x(t) = Ad*x(t-dt)+Bd*u(t)}',newline,'{\color{gray}\bf\fontsize{12}y(t) = Cd*x(t-dt)+Dd*u(t)}'], 'texmode','on');
  Discrete State-Space1 : Subsystem  mask{A=1, B=1, C=1, D=1, InitVec=1, dt=50e-6}
      mask prompts: InitVec "Initial condition:"; dt "Time step (s):"
      mask init:
      | % I = eye(size(A,1));
      | % INVR = I/(I-A*dt/2);
      | % Ad1 = INVR*(I+A*dt/2);
      | % Bd1 = INVR*B*dt/2;
      | % Cd1 = C*Ad1;
      | % Dd11 = C*INVR*B*dt/2+D;
      | % Dd12 = C*INVR*B*dt/2;
      | 
      |     I = eye(size(A,1));
      |     
      |     INVR = I/(I-A*dt/2);
      |     
      |     Ad = INVR*(I+A*dt/2);
      |     
      |     Bd = INVR*B;
      |     
      |     Cd = C*INVR*dt;
      |     
      |     Dd = Cd*B/2 + D;
      settings: LibrarySourceBlock=|
      | spsSynchronousMachineModel/Discrete robust/State Space Model/Discretize
      | BE or Tustin
      mask Display: disp(['{\color{red}\bf\fontsize{12}x(t) = Ad*x(t-dt)+Bd*u(t)}',newline,'{\color{gray}\bf\fontsize{12}y(t) = Cd*x(t-dt)+Dd*u(t)}'], 'texmode','on');

== system DQN_Lib/DQN2abc ==
  DQN : Inport
  th : Inport  Port=2
  DQn->ABC19 : MATLAB Function  TreatAsAtomicUnit=on  mask{N=HrmOrd}
      mask prompts: N "Harmonic order:"
  Demux46 : Demux  Outputs=6
  abc : Outport
  wires:
  Demux46/6 -> DQn->ABC19/6(Xqz)
  Demux46/5 -> DQn->ABC19/5(Xqn)
  Demux46/4 -> DQn->ABC19/4(Xqp)
  Demux46/3 -> DQn->ABC19/3(Xdz)
  Demux46/2 -> DQn->ABC19/2(Xdn)
  Demux46/1 -> DQn->ABC19/1(Xdp)
  th/1 -> DQn->ABC19/7(th)
  DQN/1 -> Demux46/1
  DQn->ABC19/1(abc) -> abc/1

== system DQN_Lib/Demux_DQNc_Mat ==
  In1 : Inport
  Sel1 : Selector  NumberOfDimensions=2  InputPortWidth=3  IndexOptions=Index vector (dialog),Select all  Indices=1:3, 1  OutputSizes=1
  Sel2 : Selector  NumberOfDimensions=2  InputPortWidth=3  IndexOptions=Index vector (dialog),Select all  Indices=4:6, 1  OutputSizes=1
  Out1 : Outport
  Out2 : Outport  Port=2
  wires:
  In1/1 -> Sel1/1, Sel2/1
  Sel1/1 -> Out1/1
  Sel2/1 -> Out2/1

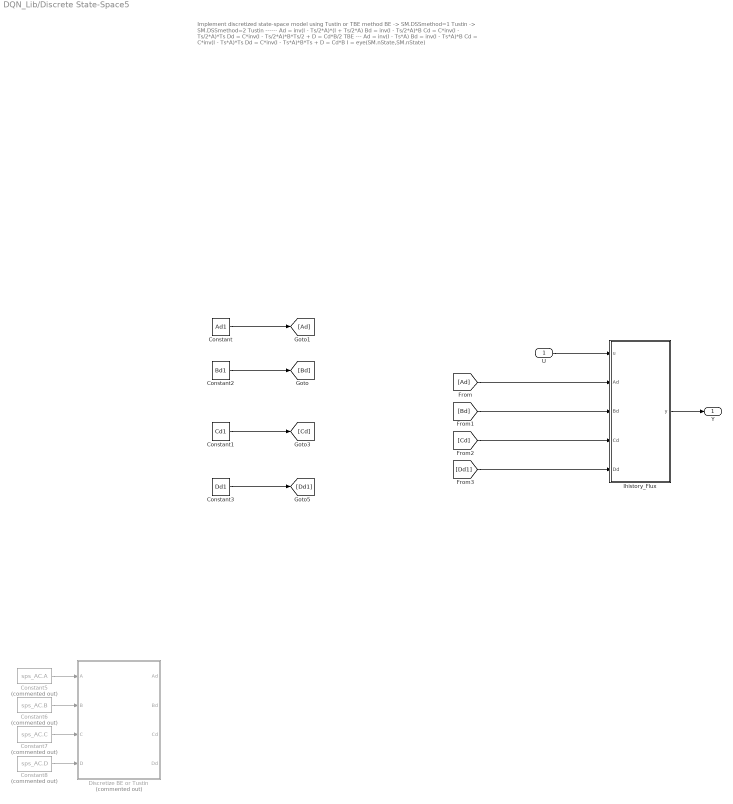
== system DQN_Lib/Discrete State-Space5 ==
  note: Implement discretized state-space model using Tustin or TBE method
      |
      | BE      -> SM.DSSmethod=1
      | Tustin  -> SM.DSSmethod=2
      |
      |
      | Tustin
      | ------
      | Ad = inv(I - Ts/2*A)*(I + Ts/2*A)
      | Bd = inv(I - Ts/2*A)*B
      | Cd = C*inv(I - Ts/2*A)*Ts
      | Dd = C*inv(I - Ts/2*A)*B*Ts/2  + D  =  Cd*B/2
      |
      | TBE
      | ---
      | Ad = inv(I - Ts*A)
      | Bd = inv(I - Ts*A)*B
      | Cd = C*inv(I - Ts*A)*Ts
      | Dd = C*inv(I - Ts*A)*B*Ts  + D  =  Cd*B
      |
      | I = eye(SM.nState,SM.nState)
  U : Inport
  Constant : Constant  Value=Ad1
  Constant1 : Constant  Value=Cd1
  Constant2 : Constant  Value=Bd1
  Constant3 : Constant  Value=Dd1
  Constant5 : Constant  Commented=on  Value=sps_AC.A
  Constant6 : Constant  Commented=on  Value=sps_AC.B
  Constant7 : Constant  Commented=on  Value=sps_AC.C
  Constant8 : Constant  Commented=on  Value=sps_AC.D
  Discretize BE or Tustin : Subsystem  Commented=on  AncestorBlock="DQN_Machines/DQN_Mac_V1/Discretize  BE or Tustin"
  Ihistory_Flux : Subsystem  AncestorBlock=DQN_Machines/DQN_Mac_V1/Ihistory_Flux
  Y : Outport
  wires:
  [Dd1] -> Ihistory_Flux/5(Dd)
  [Cd] -> Ihistory_Flux/4(Cd)
  [Bd] -> Ihistory_Flux/3(Bd)
  [Ad] -> Ihistory_Flux/2(Ad)
  Ihistory_Flux/1(y) -> Y/1
  U/1 -> Ihistory_Flux/1(u)
  Constant5/1 -> Discretize BE or Tustin/1(A)
  Constant8/1 -> Discretize BE or Tustin/4(D)
  Constant6/1 -> Discretize BE or Tustin/2(B)
  Constant7/1 -> Discretize BE or Tustin/3(C)
  Constant3/1 -> [Dd1]
  Constant1/1 -> [Cd]
  Constant2/1 -> [Bd]
  Constant/1 -> [Ad]

== system DQN_Lib/Int_DQN ==
  X_DQN : Inport
  Demux : Demux  Outputs=6
  Int_d_2N_2 : MATLAB Function  TreatAsAtomicUnit=on  mask{N=HrmOrd, dt=TimeStep, w=FreqRad, EMT=EMT, InitInt=Init, chkHrmLst=chkHrmLst, HrmLst=HrmLst}
      mask prompts: N "Order number:"; dt "Time step (s):"; w "Angular frequency (1/rad):"; InitInt "Initial conditions [6x1]:"; chkHrmLst "Only selected harmonics"; HrmLst "Harmonic list:"
  Mux51 : Mux  Inputs=[(1)*HrmOrd+1,(1)*HrmOrd+1,(1)*HrmOrd+1,(1)*HrmOrd+1,(1)*HrmOrd+1,(1)*HrmOrd+1]
  Z_DQN : Outport
  wires:
  Int_d_2N_2/6(Zqz) -> Mux51/6
  Int_d_2N_2/5(Zqn) -> Mux51/5
  Int_d_2N_2/1(Zdp) -> Mux51/1
  Int_d_2N_2/4(Zqp) -> Mux51/4
  Int_d_2N_2/2(Zdn) -> Mux51/2
  Int_d_2N_2/3(Zdz) -> Mux51/3
  Demux/6 -> Int_d_2N_2/6(Xqz)
  Demux/5 -> Int_d_2N_2/5(Xqn)
  Demux/1 -> Int_d_2N_2/1(Xdp)
  Demux/4 -> Int_d_2N_2/4(Xqp)
  Demux/2 -> Int_d_2N_2/2(Xdn)
  Demux/3 -> Int_d_2N_2/3(Xdz)
  Mux51/1 -> Z_DQN/1
  X_DQN/1 -> Demux/1

== system DQN_Lib/Int_DQN_fdbk ==
  X_DQN : Inport
  Demux : Demux  Outputs=6
  Int_d_2N_2 : MATLAB Function  TreatAsAtomicUnit=on  mask{N=HrmOrd, dt=TimeStep, w=FreqRad, SW=swFeed, R=R, iL=iL}
      mask prompts: N "Order number:"; dt "Time step (s):"; w "Angular frequency (1/rad):"; SW "Enable feedback"; R "Feedback parameter (Kr):"; iL "Integrator parameter (Kl):"
  Mux51 : Mux  Inputs=[(1)*HrmOrd+1,(1)*HrmOrd+1,(1)*HrmOrd+1,(1)*HrmOrd+1,(1)*HrmOrd+1,(1)*HrmOrd+1]
  Z_DQN : Outport
  wires:
  X_DQN/1 -> Demux/1
  Mux51/1 -> Z_DQN/1
  Demux/3 -> Int_d_2N_2/3(Xdz)
  Demux/2 -> Int_d_2N_2/2(Xdn)
  Demux/4 -> Int_d_2N_2/4(Xqp)
  Demux/1 -> Int_d_2N_2/1(Xdp)
  Demux/5 -> Int_d_2N_2/5(Xqn)
  Demux/6 -> Int_d_2N_2/6(Xqz)
  Int_d_2N_2/3(Zdz) -> Mux51/3
  Int_d_2N_2/2(Zdn) -> Mux51/2
  Int_d_2N_2/4(Zqp) -> Mux51/4
  Int_d_2N_2/1(Zdp) -> Mux51/1
  Int_d_2N_2/5(Zqn) -> Mux51/5
  Int_d_2N_2/6(Zqz) -> Mux51/6

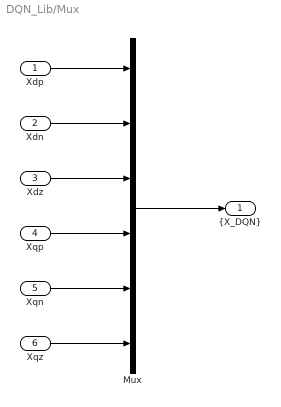
== system DQN_Lib/Mux ==
  Xdp : Inport
  Xdn : Inport  Port=2
  Xdz : Inport  Port=3
  Xqp : Inport  Port=4
  Xqn : Inport  Port=5
  Xqz : Inport  Port=6
  Mux : Mux  Inputs=[N+1, N+1, N+1, N+1, N+1, N+1]
  "{X_DQN}" : Outport
  wires:
  Xqz/1 -> Mux/6
  Xqn/1 -> Mux/5
  Xqp/1 -> Mux/4
  Xdz/1 -> Mux/3
  Xdn/1 -> Mux/2
  Xdp/1 -> Mux/1
  Mux/1 -> "{X_DQN}"/1

== system DQN_Lib/Mux_DQNc_Mat ==
  In1 : Inport
  In2 : Inport  Port=2
  Mux : Concatenate  Mode=Multidimensional array  ConcatenateDimension=nrOut
  Out1 : Outport
  wires:
  In1/1 -> Mux/1
  In2/1 -> Mux/2
  Mux/1 -> Out1/1

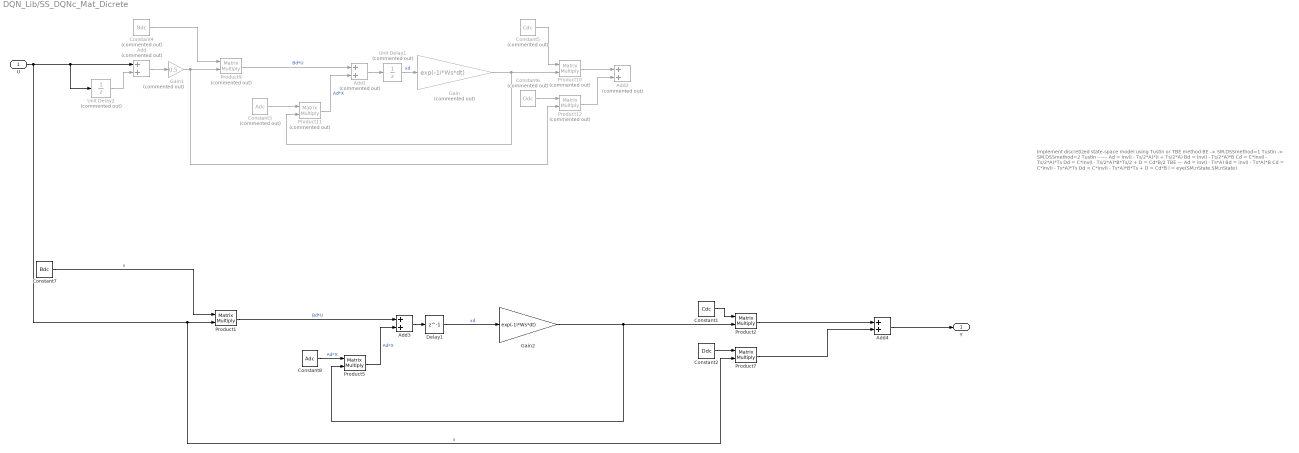
== system DQN_Lib/SS_DQNc_Mat_Dicrete ==
  note: Implement discretized state-space model using Tustin or TBE method
      |
      | BE      -> SM.DSSmethod=1
      | Tustin  -> SM.DSSmethod=2
      |
      |
      | Tustin
      | ------
      | Ad = inv(I - Ts/2*A)*(I + Ts/2*A)
      | Bd = inv(I - Ts/2*A)*B
      | Cd = C*inv(I - Ts/2*A)*Ts
      | Dd = C*inv(I - Ts/2*A)*B*Ts/2  + D  =  Cd*B/2
      |
      | TBE
      | ---
      | Ad = inv(I - Ts*A)
      | Bd = inv(I - Ts*A)*B
      | Cd = C*inv(I - Ts*A)*Ts
      | Dd = C*inv(I - Ts*A)*B*Ts  + D  =  Cd*B
      |
      | I = eye(SM.nState,SM.nState)
  U : Inport
  Add : Sum  Commented=on
  Add1 : Sum  Commented=on
  Add2 : Sum  Commented=on
  Add3 : Sum
  Add4 : Sum
  Constant1 : Constant  Value=Cdc
  Constant2 : Constant  Value=Ddc
  Constant3 : Constant  Commented=on  Value=Adc
  Constant4 : Constant  Commented=on  Value=Bdc
  Constant5 : Constant  Commented=on  Value=Cdc
  Constant6 : Constant  Commented=on  Value=Ddc
  Constant7 : Constant  Value=Bdc
  Constant8 : Constant  Value=Adc
  Delay1 : Delay  DelayLength=1  SampleTime=dt
  Gain : Gain  Commented=on  Gain=exp(-1i*Ws*dt)
  Gain1 : Gain  Commented=on  Gain=0.5
  Gain2 : Gain  Gain=exp(-1i*Ws*dt)
  Product{1..2,5,7} (4 alike) : Product  Multiplication=Matrix(*)  SaturateOnIntegerOverflow=on  OutDataTypeStr=Inherit: Same as first input
  Product{9..12} (4 alike) : Product  Commented=on  Multiplication=Matrix(*)  SaturateOnIntegerOverflow=on  OutDataTypeStr=Inherit: Same as first input
  Unit Delay1 : UnitDelay  Commented=on  InitialCondition=InitVec_c  SampleTime=dt  HasFrameUpgradeWarning=on
  Unit Delay2 : UnitDelay  Commented=on  SampleTime=dt  HasFrameUpgradeWarning=on
  Y : Outport
  wires:
  Product12/1 -> Add2/2
  Constant3/1 -> Product11/1
  Constant6/1 -> Product12/1
  Product10/1 -> Add2/1
  Unit Delay1/1 -> Gain/1  "xd"
  Product9/1 -> Add1/1  "Bd*U"
  Add1/1 -> Unit Delay1/1
  Product11/1 -> Add1/2  "Ad*X"
  Gain1/1 -> Product12/2, Product9/2
  Constant4/1 -> Product9/1
  Unit Delay2/1 -> Add/2
  Add/1 -> Gain1/1
  Constant5/1 -> Product10/1
  Gain/1 -> Product11/2, Product10/2
  Delay1/1 -> Gain2/1  "xd"
  Constant8/1 -> Product5/1  "Ad*X"
  Product5/1 -> Add3/2  "Ad*X"
  Add4/1 -> Y/1
  Product2/1 -> Add4/1
  Constant1/1 -> Product2/1
  Constant7/1 -> Product1/1  "u"
  Product1/1 -> Add3/1  "Bd*U"
  Add3/1 -> Delay1/1
  U/1 -> Product7/2, Product1/2, Unit Delay2/1, Add/1  "u"
  Product7/1 -> Add4/2
  Constant2/1 -> Product7/1
  Gain2/1 -> Product5/2, Product2/2

== system DQN_Lib/SS_DelayPrediction ==
  in : Inport
  F2 : Gain  Gain=2  SaturateOnIntegerOverflow=on  OutDataTypeStr=Inherit: Same as input  ParamDataTypeStr=Inherit: Same as input
  Sum1 : Sum  Inputs=+-  InputSameDT=on  SaturateOnIntegerOverflow=on  OutDataTypeStr=Inherit: Same as first input
  dw_delay : UnitDelay  InitialCondition=Zpnz_old  SampleTime=Ts  HasFrameUpgradeWarning=on
  dw_predict : UnitDelay  InitialCondition=Zpnz_old  SampleTime=Ts  HasFrameUpgradeWarning=on
  dw : Outport  VectorParamsAs1DForOutWhenUnconnected=off
  wires:
  dw_delay/1 -> dw_predict/1, F2/1
  in/1 -> dw_delay/1
  dw_predict/1 -> Sum1/2
  F2/1 -> Sum1/1
  Sum1/1 -> dw/1

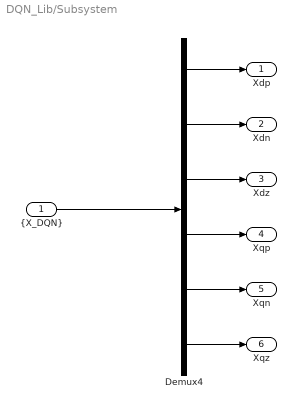
== system DQN_Lib/Subsystem ==
  "{X_DQN}" : Inport
  Demux4 : Demux  Outputs=[N+1, N+1, N+1, N+1, N+1, N+1]
  Xdp : Outport
  Xdn : Outport  Port=2
  Xdz : Outport  Port=3
  Xqp : Outport  Port=4
  Xqn : Outport  Port=5
  Xqz : Outport  Port=6
  wires:
  Demux4/6 -> Xqz/1
  Demux4/5 -> Xqn/1
  Demux4/4 -> Xqp/1
  Demux4/3 -> Xdz/1
  Demux4/2 -> Xdn/1
  Demux4/1 -> Xdp/1
  "{X_DQN}"/1 -> Demux4/1

== system DQN_Lib/Subsystem1 ==
  abc : Inport
  th : Inport  Port=2
  DQN Mux : MATLAB Function  TreatAsAtomicUnit=on  mask{N=1}
      mask prompts: N "Harmonic order:"
  Mux : Mux  Inputs=[1, 1, 1, 1, 1, 1]
  Mux1 : Mux  Inputs=2
  abc-->DQN : DQN_Lib_bak/abc-->DQN  H=HrmOrd  f=Freq  Ts=Ts
  DQN : Outport
  wires:
  Mux/1 -> Mux1/2
  Mux1/1 -> DQN Mux/1(u)
  abc-->DQN/1 -> Mux1/1
  DQN Mux/1(y) -> DQN/1
  abc-->DQN/7 -> Mux/6
  abc-->DQN/6 -> Mux/5
  abc-->DQN/5 -> Mux/4
  abc-->DQN/4 -> Mux/3
  abc-->DQN/3 -> Mux/2
  abc-->DQN/2 -> Mux/1
  abc/1 -> abc-->DQN/1
  th/1 -> abc-->DQN/2

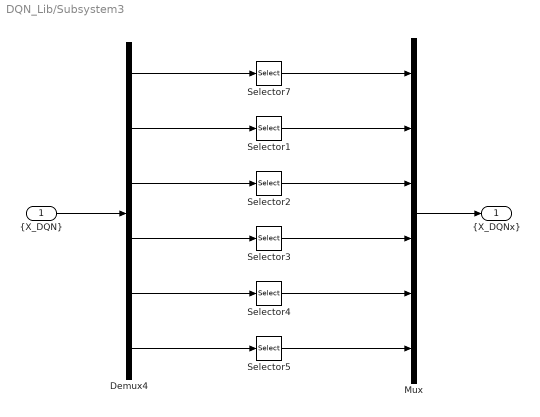
== system DQN_Lib/Subsystem3 ==
  "{X_DQN}" : Inport
  Demux4 : Demux  Outputs=[HOI+1,HOI+1,HOI+1,HOI+1,HOI+1,HOI+1]
  Mux : Mux  Inputs=[HOO+1,HOO+1,HOO+1,HOO+1,HOO+1,HOO+1]
  Selector{1..5,7} (6 alike) : Selector  InputPortWidth=HOI+1  IndexOptions=Index vector (dialog)  Indices=[1:HOO+1]  OutputSizes=1
  "{X_DQNx}" : Outport
  wires:
  Selector5/1 -> Mux/6
  Demux4/6 -> Selector5/1
  Selector4/1 -> Mux/5
  Demux4/5 -> Selector4/1
  Selector3/1 -> Mux/4
  Demux4/4 -> Selector3/1
  Selector2/1 -> Mux/3
  Demux4/3 -> Selector2/1
  Demux4/2 -> Selector1/1
  Selector1/1 -> Mux/2
  Demux4/1 -> Selector7/1
  Selector7/1 -> Mux/1
  Mux/1 -> "{X_DQNx}"/1
  "{X_DQN}"/1 -> Demux4/1

== system DQN_Lib/Subsystem4 ==
  In1 : Inport
  In2 : Inport  Port=2
  Demux : Demux  Outputs=6
  S-Function : S-Function  FunctionName=sDQNabc  SFunctionDeploymentMode=off  EnableBusSupport=off
  Out1 : Outport
  wires:
  In1/1 -> Demux/1
  In2/1 -> S-Function/7
  Demux/3 -> S-Function/3
  Demux/1 -> S-Function/1
  S-Function/1 -> Out1/1
  Demux/2 -> S-Function/2
  Demux/6 -> S-Function/6
  Demux/4 -> S-Function/4
  Demux/5 -> S-Function/5

== system DQN_Lib/sAdd_DQN ==
  In1 : Inport
  In2 : Inport  Port=2
  Demux : Demux  Outputs=6
  Demux7 : Demux  Outputs=6
  Mux7 : Mux  Inputs=[HRM+1,HRM+1,HRM+1,HRM+1,HRM+1,HRM+1]
  S-Function : S-Function  FunctionName=sAddDQN  Parameters=HRM  SFunctionDeploymentMode=off  EnableBusSupport=off  mask{HRM=HRM}
      mask prompts: HRM "Harmonic order:"
  Out1 : Outport
  wires:
  In1/1 -> Demux/1
  Demux/1 -> S-Function/1
  Demux7/2 -> S-Function/8
  Demux7/6 -> S-Function/12
  Demux/5 -> S-Function/5
  Demux7/4 -> S-Function/10
  Demux7/1 -> S-Function/7
  Demux/4 -> S-Function/4
  Demux7/3 -> S-Function/9
  Mux7/1 -> Out1/1
  Demux/6 -> S-Function/6
  In2/1 -> Demux7/1
  Demux/2 -> S-Function/2
  S-Function/2 -> Mux7/2
  Demux/3 -> S-Function/3
  S-Function/1 -> Mux7/1
  S-Function/5 -> Mux7/5
  Demux7/5 -> S-Function/11
  S-Function/3 -> Mux7/3
  S-Function/4 -> Mux7/4
  S-Function/6 -> Mux7/6

== system DQN_Lib/sDQN2abc ==
  "{DQN}" : Inport
  th : Inport  Port=2
  Demux : Demux  Outputs=6
  S-Function : S-Function  FunctionName=sDQNabcN  Parameters=HRM  SFunctionDeploymentMode=off  EnableBusSupport=off
  abc : Outport
  wires:
  "{DQN}"/1 -> Demux/1
  Demux/6 -> S-Function/6
  Demux/5 -> S-Function/5
  Demux/4 -> S-Function/4
  Demux/3 -> S-Function/3
  Demux/2 -> S-Function/2
  Demux/1 -> S-Function/1
  th/1 -> S-Function/7
  S-Function/1 -> abc/1

== system DQN_Lib/sInt_DQN ==
  In1 : Inport
  Demux : Demux  Outputs=[HRM+1,HRM+1,HRM+1,HRM+1,HRM+1,HRM+1]
  Mux1 : Mux  Inputs=[HRM+1,HRM+1,HRM+1,HRM+1,HRM+1,HRM+1]
  S-Function : S-Function  FunctionName=sIntDQN  Parameters=HRM Ts Ws HrmSeq  SFunctionDeploymentMode=off  EnableBusSupport=off
  Out1 : Outport
  wires:
  Mux1/1 -> Out1/1
  In1/1 -> Demux/1
  S-Function/3 -> Mux1/3
  S-Function/5 -> Mux1/5
  S-Function/2 -> Mux1/2
  S-Function/4 -> Mux1/4
  Demux/4 -> S-Function/4
  S-Function/6 -> Mux1/6
  Demux/5 -> S-Function/5
  Demux/1 -> S-Function/1
  Demux/2 -> S-Function/2
  Demux/6 -> S-Function/6
  S-Function/1 -> Mux1/1
  Demux/3 -> S-Function/3

== system DQN_Lib/sInt_DQN_fdbk ==
  In1 : Inport
  Demux : Demux  Outputs=[HRM+1,HRM+1,HRM+1,HRM+1,HRM+1,HRM+1]
  Mux1 : Mux  Inputs=[HRM+1,HRM+1,HRM+1,HRM+1,HRM+1,HRM+1]
  S-Function : S-Function  FunctionName=sIntDQNfdbk  Parameters=HRM Ts Ws HrmSeq swFeed R iL  SFunctionDeploymentMode=off  EnableBusSupport=off
  Out1 : Outport
  wires:
  Demux/3 -> S-Function/3
  S-Function/1 -> Mux1/1
  Demux/6 -> S-Function/6
  Demux/2 -> S-Function/2
  Demux/1 -> S-Function/1
  Demux/5 -> S-Function/5
  S-Function/6 -> Mux1/6
  Demux/4 -> S-Function/4
  S-Function/4 -> Mux1/4
  S-Function/2 -> Mux1/2
  S-Function/5 -> Mux1/5
  S-Function/3 -> Mux1/3
  In1/1 -> Demux/1
  Mux1/1 -> Out1/1

== system DQN_Lib/sMult_DQN ==
  In1 : Inport
  In2 : Inport  Port=2
  Demux : Demux  Outputs=6
  Demux7 : Demux  Outputs=6
  Mux7 : Mux  Inputs=[(HrmDbl+1)*HRM+1,(HrmDbl+1)*HRM+1,(HrmDbl+1)*HRM+1,(HrmDbl+1)*HRM+1,(HrmDbl+1)*HRM+1,(HrmDbl+1)*HRM+1]
  S-Function : S-Function  FunctionName=sMultDQN  Parameters=HRM chkHrm  SFunctionDeploymentMode=off  EnableBusSupport=off  mask{HRM=HRM, chkHrm=HrmOpt}
      mask prompts: HRM "Harmonic order:"; chkHrm "Double harmonic:"
  Out1 : Outport
  wires:
  In1/1 -> Demux/1
  Demux/1 -> S-Function/1
  Demux7/2 -> S-Function/8
  Demux7/6 -> S-Function/12
  Demux/5 -> S-Function/5
  Demux7/4 -> S-Function/10
  Demux7/1 -> S-Function/7
  Demux/4 -> S-Function/4
  Demux7/3 -> S-Function/9
  Mux7/1 -> Out1/1
  Demux/6 -> S-Function/6
  In2/1 -> Demux7/1
  Demux/2 -> S-Function/2
  S-Function/2 -> Mux7/2
  Demux/3 -> S-Function/3
  S-Function/1 -> Mux7/1
  S-Function/5 -> Mux7/5
  Demux7/5 -> S-Function/11
  S-Function/3 -> Mux7/3
  S-Function/4 -> Mux7/4
  S-Function/6 -> Mux7/6

== system DQN_Lib/sMult_DQN_old ==
  In1 : Inport
  In2 : Inport  Port=2
  Demux : Demux  Outputs=6
  Demux7 : Demux  Outputs=6
  Mux7 : Mux  Inputs=[(HrmDbl+1)*HrmOrd+1,(HrmDbl+1)*HrmOrd+1,(HrmDbl+1)*HrmOrd+1,(HrmDbl+1)*HrmOrd+1,(HrmDbl+1)*HrmOrd+1,(HrmDbl+1)*HrmOrd+1]
  S-Function : S-Function  FunctionName=sMultDQN  Parameters=HRM  SFunctionDeploymentMode=off  EnableBusSupport=off  mask{HRM=HrmOrd}
      mask prompts: HRM "Harmonic order:"
  Out1 : Outport
  wires:
  S-Function/3 -> Mux7/3
  S-Function/2 -> Mux7/2
  Demux7/5 -> S-Function/11
  Demux/5 -> S-Function/5
  Demux/3 -> S-Function/3
  Demux7/1 -> S-Function/7
  Demux/6 -> S-Function/6
  Demux/1 -> S-Function/1
  Demux/4 -> S-Function/4
  S-Function/4 -> Mux7/4
  Demux7/6 -> S-Function/12
  Demux7/3 -> S-Function/9
  Demux7/2 -> S-Function/8
  Demux7/4 -> S-Function/10
  Demux/2 -> S-Function/2
  S-Function/6 -> Mux7/6
  S-Function/1 -> Mux7/1
  In2/1 -> Demux7/1
  S-Function/5 -> Mux7/5
  In1/1 -> Demux/1
  Mux7/1 -> Out1/1

== system DQN_Lib/sSumDQN ==
  In1 : Inport
  Demux18 : Demux  Outputs=[HrmOrd+1,HrmOrd+1,HrmOrd+1,HrmOrd+1,HrmOrd+1,HrmOrd+1]
  Mux26 : Mux  Inputs=[HrmOrd+1,HrmOrd+1,HrmOrd+1,HrmOrd+1,HrmOrd+1,HrmOrd+1]
  S-Function : S-Function  FunctionName=sSumDQN  Parameters=HrmOrd  SFunctionDeploymentMode=off  EnableBusSupport=off
  Out1 : Outport
  wires:
  Mux26/1 -> Out1/1
  S-Function/5 -> Mux26/5  "(HrmDbl+1)*HRM+1"
  S-Function/4 -> Mux26/4  "(HrmDbl+1)*HRM+1"
  Demux18/1 -> S-Function/1
  S-Function/3 -> Mux26/3  "(HrmDbl+1)*HRM+1"
  Demux18/6 -> S-Function/6
  S-Function/2 -> Mux26/2  "(HrmDbl+1)*HRM+1"
  In1/1 -> Demux18/1
  S-Function/6 -> Mux26/6  "(HrmDbl+1)*HRM+1]"
  Demux18/4 -> S-Function/4
  Demux18/2 -> S-Function/2
  Demux18/5 -> S-Function/5
  Demux18/3 -> S-Function/3
  S-Function/1 -> Mux26/1  "[(HrmDbl+1)*HRM+1"
